simulink model "Lab1_P"  (R2019a)
settings: Solver=VariableStepAuto  StartTime=0.0  StopTime=1000  RelTol=1e-3
undefined symbols (not defined in the file or in its folder): G1, G2
settings Model: Creator=Gabe Casciano  LastModifiedBy=Gabe Casciano

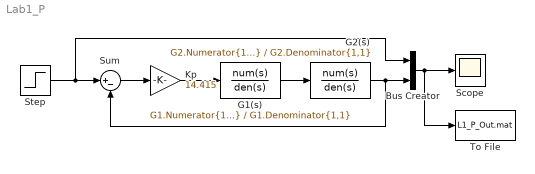
== system Lab1_P ==
  Bus Creator : BusCreator  Inputs=2
  G1(s) : TransferFcn  Numerator=G1.Numerator{1,1}  Denominator=G1.Denominator{1,1}
  G2(s) : TransferFcn  Numerator=G2.Numerator{1,1}  Denominator=G2.Denominator{1,1}
  Kp : Gain  Gain=14.415
  Scope : Scope
  Step : Step  Time=0  SampleTime=0
  Sum : Sum  Inputs=|+-
  To File : ToFile  Filename=L1_P_Out.mat  MatrixName=L1_P_Out  SaveFormat=Timeseries
  wires:
  Sum/1 -> Kp/1
  Kp/1 -> G1(s)/1
  G1(s)/1 -> G2(s)/1
  Step/1 -> Sum/1, Bus Creator/1
  Bus Creator/1 -> To File/1, Scope/1
  G2(s)/1 -> Sum/2, Bus Creator/2
